simulink model "FixedWingModel"  (R2021a)
settings: configuration reference "ctrlConfigSet" (kept outside this file)
libraries: simulink x1
settings Model: DataDictionary=pathFollowingData.sldd  Creator=The MathWorks, Inc.  LastModifiedBy=hgu8
settings ConfigSetRef: SourceName=ctrlConfigSet

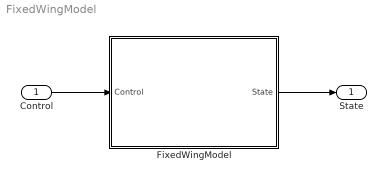
== system FixedWingModel ==
  Control : Inport  OutDataTypeStr=Bus: FixedWingControlBus2  BusOutputAsStruct=on
  FixedWingModel : Subsystem  Variant=on
  State : Outport  OutDataTypeStr=Bus: FixedWingStateBus  VectorParamsAs1DForOutWhenUnconnected=off  BusOutputAsStruct=on
  wires:
  FixedWingModel/1(State) -> State/1
  Control/1 -> FixedWingModel/1(Control)

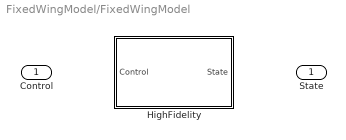
== system FixedWingModel/FixedWingModel ==
  Control : Inport
  HighFidelity : Subsystem  VariantControl=useHighFidelity == 1
  State : Outport  VectorParamsAs1DForOutWhenUnconnected=off

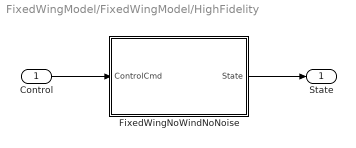
== system FixedWingModel/FixedWingModel/HighFidelity ==
  Control : Inport
  FixedWingNoWindNoNoise : Subsystem
  State : Outport  VectorParamsAs1DForOutWhenUnconnected=off
  wires:
  FixedWingNoWindNoNoise/1(State) -> State/1
  Control/1 -> FixedWingNoWindNoNoise/1(ControlCmd)

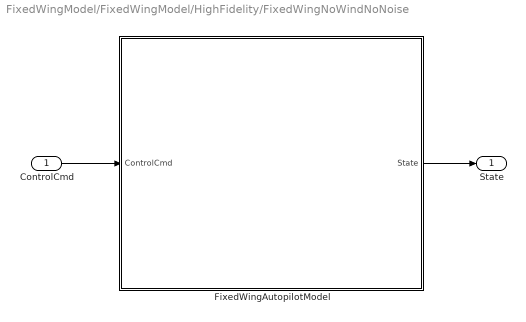
== system FixedWingModel/FixedWingModel/HighFidelity/FixedWingNoWindNoNoise ==
  ControlCmd : Inport  OutDataTypeStr=Bus: FixedWingControlBus2
  FixedWingAutopilotModel : Subsystem
  State : Outport  VectorParamsAs1DForOutWhenUnconnected=off
  wires:
  ControlCmd/1 -> FixedWingAutopilotModel/1(ControlCmd)
  FixedWingAutopilotModel/1(State) -> State/1

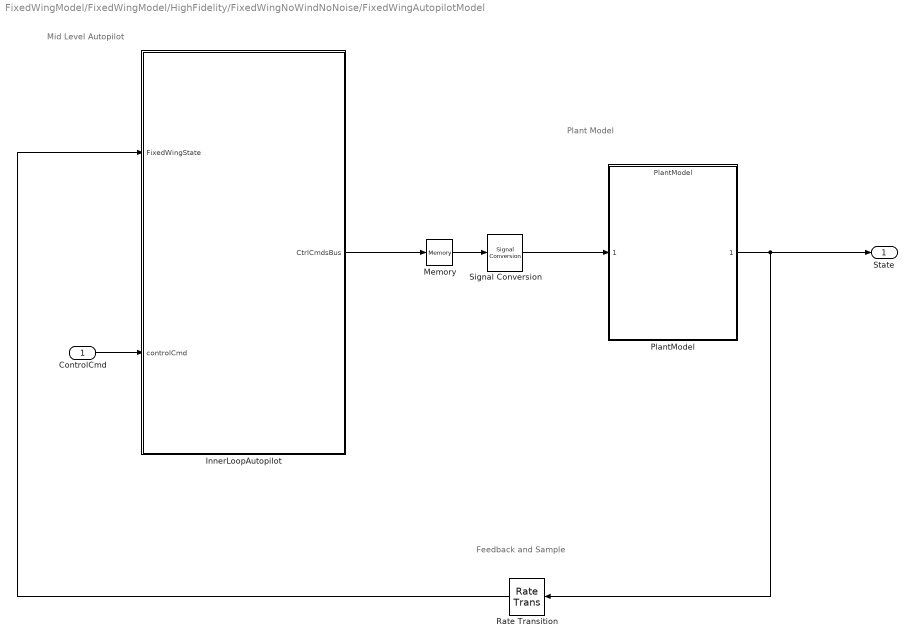
== system FixedWingModel/FixedWingModel/HighFidelity/FixedWingNoWindNoNoise/FixedWingAutopilotModel ==
  note: Mid Level Autopilot
  note: Plant Model
  note: Feedback and Sample
  ControlCmd : Inport  OutDataTypeStr=Bus: FixedWingControlBus2
  InnerLoopAutopilot : Subsystem  TreatAsAtomicUnit=on
  Memory : Memory
  PlantModel : ModelReference  ModelNameDialog=PlantModel.slx  SimulationMode=Normal  ModelReferenceVersion=3.23
  Rate Transition : RateTransition  OutPortSampleTime=ap.apSampleTime
  Signal Conversion : SignalConversion  ConversionOutput=Nonvirtual bus  OutDataTypeStr=Bus: ctrlCmdsBus  OverrideOpt=off
  State : Outport  OutDataTypeStr=Bus: FixedWingStateBus
  wires:
  ControlCmd/1 -> InnerLoopAutopilot/2(controlCmd)
  InnerLoopAutopilot/1(CtrlCmdsBus) -> Memory/1
  Rate Transition/1 -> InnerLoopAutopilot/1(FixedWingState)
  Signal Conversion/1 -> PlantModel/1
  Memory/1 -> Signal Conversion/1
  PlantModel/1 -> State/1, Rate Transition/1

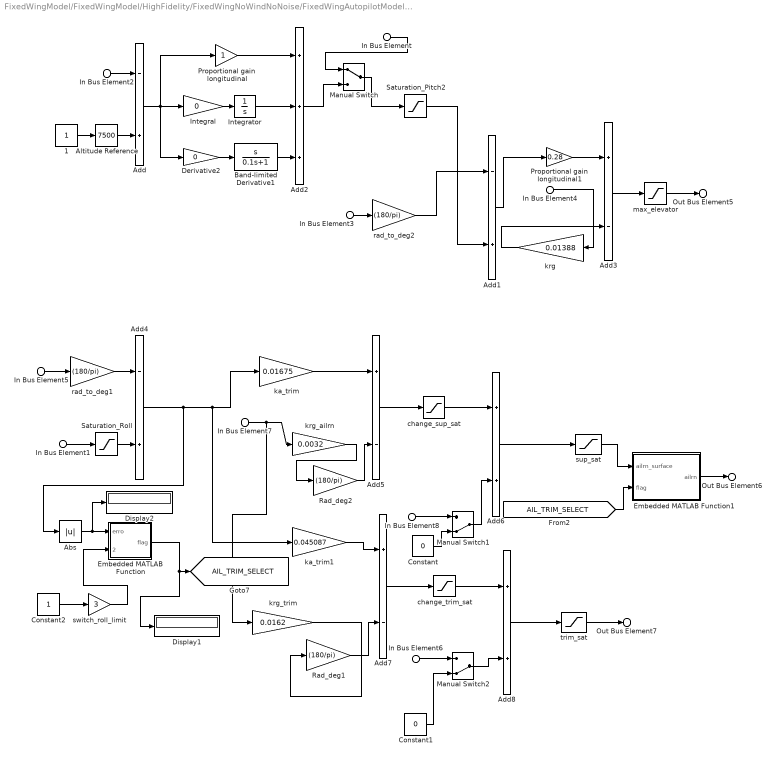
== system FixedWingModel/FixedWingModel/HighFidelity/FixedWingNoWindNoNoise/FixedWingAutopilotModel/InnerLoopAutopilot ==
  In Bus Element6 : Inport  PortName=FixedWingState  Element=Aileron_Trim
  In Bus Element2 : Inport  PortName=FixedWingState  Element=Altitude
  In Bus Element3 : Inport  PortName=FixedWingState  Element=PitchAngle
  In Bus Element4 : Inport  PortName=FixedWingState  Element=q
  In Bus Element5 : Inport  PortName=FixedWingState  Element=RollAngle
  In Bus Element7 : Inport  PortName=FixedWingState  Element=P
  In Bus Element8 : Inport  PortName=FixedWingState  Element=Aileron
  In Bus Element : Inport  Port=2  PortName=controlCmd  Element=Pitch_Ref
  In Bus Element1 : Inport  Port=2  PortName=controlCmd  Element=Roll_Ref
  " 1" : Constant
  Abs : Abs
  Add : Sum  Inputs=-+
  Add1 : Sum  Inputs=-+
  Add2 : Sum  Inputs=+++
  Add3 : Sum  Inputs=+-
  Add4 : Sum  Inputs=-+
  Add5 : Sum  Inputs=+-
  Add6 : Sum
  Add7 : Sum  Inputs=+-
  Add8 : Sum
  Altitude Reference : simulink/Math Operations/Slider Gain  gain=7500  low=5000  high=10000
  Band-limited Derivative1 : TransferFcn  Numerator=[1 0]  Denominator=[0.1 1]
  Constant : Constant  Value=0
  Constant1 : Constant  Value=0
  Constant2 : Constant
  Derivative2 : Gain  Gain=0  SaturateOnIntegerOverflow=on  OutDataTypeStr=Inherit: Same as input  ParamDataTypeStr=Inherit: Same as input
  Display1 : Display
  Display2 : Display
  Embedded MATLAB Function : MATLAB Function  TreatAsAtomicUnit=on
  Embedded MATLAB Function1 : MATLAB Function  TreatAsAtomicUnit=on
  Integral : Gain  Gain=0  SaturateOnIntegerOverflow=on  OutDataTypeStr=Inherit: Same as input  ParamDataTypeStr=Inherit: Same as input
  Integrator : Integrator
  Manual Switch : ManualSwitch
  Manual Switch1 : ManualSwitch  CurrentSetting=0
  Manual Switch2 : ManualSwitch  CurrentSetting=0
  Proportional gain longitudinal : Gain
  Proportional gain longitudinal1 : Gain  Gain=0.28
  Rad_deg1 : Gain  Gain=(180/pi)
  Rad_deg2 : Gain  Gain=(180/pi)
  Saturation_Pitch2 : Saturate  UpperLimit=20  LowerLimit=-20
  Saturation_Roll : Saturate  UpperLimit=20  LowerLimit=-20
  change_sup_sat : Saturate  UpperLimit=0.1  LowerLimit=-0.1
  change_trim_sat : Saturate  UpperLimit=0.1  LowerLimit=-0.1
  ka_trim : Gain  Gain=0.01675  OutDataTypeStr=Inherit: Same as input  ParamDataTypeStr=Inherit: Same as input
  ka_trim1 : Gain  Gain=0.045087  OutDataTypeStr=Inherit: Same as input  ParamDataTypeStr=Inherit: Same as input
  krg : Gain  Gain=0.01388  OutDataTypeStr=Inherit: Same as input  ParamDataTypeStr=Inherit: Same as input
  krg_ailrn : Gain  Gain=0.0032  OutDataTypeStr=Inherit: Same as input  ParamDataTypeStr=Inherit: Same as input
  krg_trim : Gain  Gain=0.0162  OutDataTypeStr=Inherit: Same as input  ParamDataTypeStr=Inherit: Same as input
  max_elevator : Saturate
  rad_to_deg1 : Gain  Gain=(180/pi)
  rad_to_deg2 : Gain  Gain=(180/pi)
  sup_sat : Saturate  UpperLimit=0.9  LowerLimit=-0.9  OutMin=-1  OutMax=1  OutDataTypeStr=double  RndMeth=Nearest
  switch_roll_limit : Gain  Gain=3
  trim_sat : Saturate  UpperLimit=1  LowerLimit=-1  OutMin=-1  OutMax=1  OutDataTypeStr=double  RndMeth=Nearest
  Out Bus Element5 : Outport  PortName=CtrlCmdsBus  Element=elevator
  Out Bus Element6 : Outport  PortName=CtrlCmdsBus  Element=aileron
  Out Bus Element7 : Outport  PortName=CtrlCmdsBus  Element=aileronTrim
  tag scope: AIL_TRIM_SELECT=global
  wires:
  " 1"/1 -> Altitude Reference/1
  rad_to_deg2/1 -> Add1/1
  Altitude Reference/1 -> Add/2
  Saturation_Roll/1 -> Add4/2
  rad_to_deg1/1 -> Add4/1
  In Bus Element/1 -> Manual Switch/1
  In Bus Element1/1 -> Saturation_Roll/1
  In Bus Element5/1 -> rad_to_deg1/1
  In Bus Element7/1 -> krg_trim/1, krg_ailrn/1
  In Bus Element8/1 -> Manual Switch1/1
  In Bus Element6/1 -> Manual Switch2/1
  In Bus Element2/1 -> Add/1
  In Bus Element3/1 -> rad_to_deg2/1
  In Bus Element4/1 -> krg/1
  Derivative2/1 -> Band-limited Derivative1/1
  Proportional gain longitudinal1/1 -> Add3/1
  krg/1 -> Add3/2
  Add1/1 -> Proportional gain longitudinal1/1
  Integrator/1 -> Add2/2
  Add3/1 -> max_elevator/1
  Saturation_Pitch2/1 -> Add1/2
  Integral/1 -> Integrator/1
  max_elevator/1 -> Out Bus Element5/1
  Manual Switch/1 -> Saturation_Pitch2/1
  Band-limited Derivative1/1 -> Add2/3
  Add2/1 -> Manual Switch/2
  Add/1 -> Proportional gain longitudinal/1, Integral/1, Derivative2/1
  Proportional gain longitudinal/1 -> Add2/1
  Embedded MATLAB Function1/1(ailrn) -> Out Bus Element6/1
  Add6/1 -> sup_sat/1
  krg_ailrn/1 -> Rad_deg2/1
  Constant/1 -> Manual Switch1/2
  Manual Switch1/1 -> Add6/2
  Abs/1 -> Embedded MATLAB Function/1(erro), Display2/1
  Constant1/1 -> Manual Switch2/2
  Manual Switch2/1 -> Add8/2
  Rad_deg1/1 -> Add7/2
  Embedded MATLAB Function/1(flag) -> Display1/1, [AIL_TRIM_SELECT]
  Constant2/1 -> switch_roll_limit/1
  Add4/1 -> Abs/1, ka_trim/1, ka_trim1/1
  krg_trim/1 -> Rad_deg1/1
  change_sup_sat/1 -> Add6/1
  change_trim_sat/1 -> Add8/1
  ka_trim/1 -> Add5/1
  Add5/1 -> change_sup_sat/1
  Rad_deg2/1 -> Add5/2
  trim_sat/1 -> Out Bus Element7/1
  switch_roll_limit/1 -> Embedded MATLAB Function/2(erro_max)
  ka_trim1/1 -> Add7/1
  Add7/1 -> change_trim_sat/1
  sup_sat/1 -> Embedded MATLAB Function1/1(ailrn_surface)
  Add8/1 -> trim_sat/1
  [AIL_TRIM_SELECT] -> Embedded MATLAB Function1/2(flag)

== matlab function FixedWingModel/HighFidelity/FixedWingNoWindNoNoise/FixedWingAutopilotModel/InnerLoopAutopilot/Embedded MATLAB Function ==
  data: flag output; erro input; erro_max input
function flag = fcn(erro,erro_max)
% This block supports the Embedded MATLAB subset.
% See the help menu for details. 
if(erro<erro_max)
    flag = 1;
else
    flag = 2;
end;

== matlab function FixedWingModel/HighFidelity/FixedWingNoWindNoNoise/FixedWingAutopilotModel/InnerLoopAutopilot/Embedded MATLAB Function1 ==
  data: ailrn_surface input; flag input; ailrn output
function ailrn   = fcn_elev(ailrn_surface,flag)
% This block supports the Embedded MATLAB subset.
% See the help menu for details. 

if(flag == 1)
   
    ailrn = 0;
else
  
   ailrn = ailrn_surface;
end
